simulink model "ShipSim2"  (R2022a)
settings: Solver=VariableStepAuto  StartTime=0.0  StopTime=50000.0  RelTol=1e-3
libraries: mssSimulink x1
settings Model: Creator=ADMIN  LastModifiedBy=ADMIN

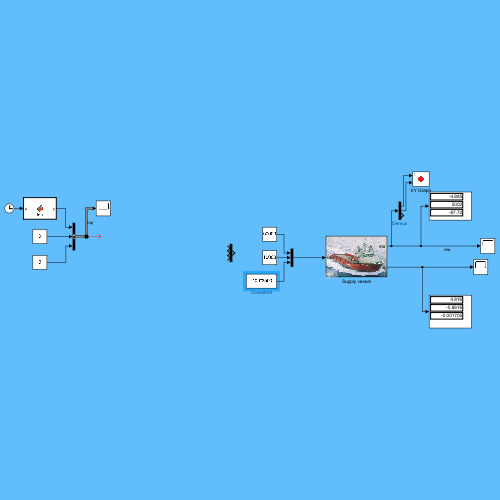
[thumbnail: Simulink's stored preview of the top-level diagram]
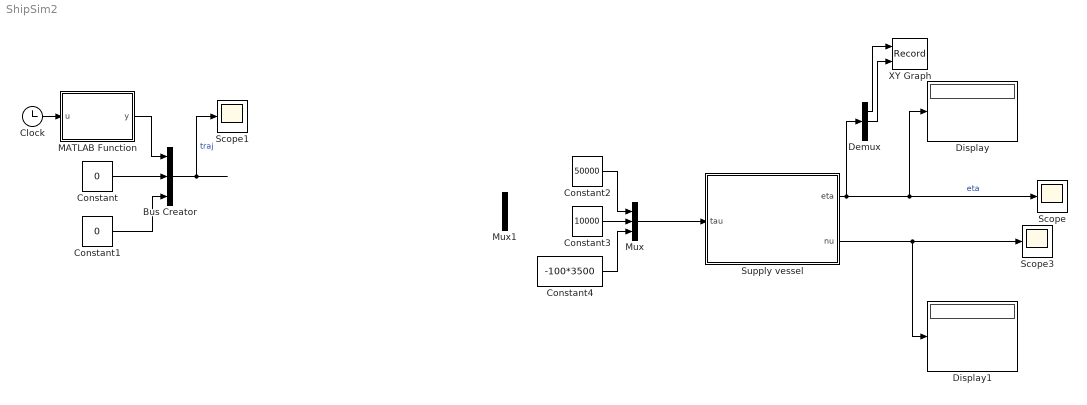
== system ShipSim2 ==
  Bus Creator : BusCreator  Inputs=3
  Clock : Clock
      settings: Decimation=50
  Constant : Constant  Value=0
  Constant1 : Constant  Value=0
  Constant2 : Constant  Value=50000
  Constant3 : Constant  Value=10000
  Constant4 : Constant  Value=-100*3500
  Demux : Demux  Outputs=3
  Display : Display
  Display1 : Display
  MATLAB Function : MATLAB Function  TreatAsAtomicUnit=on
  Mux : Mux  Inputs=3
  Mux1 : Mux  Inputs=3
  Scope : Scope
  Scope1 : Scope
  Scope3 : Scope
  Supply vessel : Subsystem  AncestorBlock=mssSimulink/Marine craft models/Supply vessel  mask(Supply Vessel (surge, sway and yaw)){D=[5.0242e4 0 0; 0 2.7229e5 -4.3933e6; 0 -4.3933e6 4.1894e8], Minv=inv( [5.3122e6 0 0; 0 8.2831e6 0; 0 0 3.7454e9] )}
      mask prompts: D "Linear damping matrix: D"; Minv "Inverse inertia matrix: Minv"
      mask help:
      | DP model
      |
      | Inputs:
      |
      |    tau = 3 DOF control input vector (generalized force)
      |
      | Outputs:
      |
      |    eta = [x, y, psi]'
      |    nu  = [u, v, r]'
      mask Display:
      | image(imread('simulink/figs/supply.jpg'))
      | color('black'); port_label('output', 1, 'eta')
      | color('black'); port_label('output', 2, 'nu')
      | color('black'); port_label('input', 1, 'tau')
  XY Graph : Record  FileSettingsInternal="{\"entries\":[{\"content\":{\"excelSettings\":{\"content\":{},\"type\":\"Streamout.ExcelSettings\"}},\"type\":\"Streamout.FileSettingStorage\",\"uuid\":\"1ec113a0-ed55-4165-962c-55b1411d3cfe\"}],\"packageUris\":[\"http://schema.mathworks.com/mf0/streamout_blocks/R2020a\"],\"version\":\"1.0\"}"  Layout=[1 1]  SignalsInternal="{\"entries\":[{\"content\":{\"signals\":[{\"content\":{\"blockPath\":[\"ShipSim2/XY Graph\"],\"channel\":[],\"dimensions\":[1],\"domain\":\"ShipSim2/XY Graph\",\"lineColor\":\"#a2142f\",\"plots\":[1],\"port\":1,\"sid\":[\"\"],\"signalID\":249,\"signalName\":\"Demux:1\"},\"type\":\"RecordBlkView.Signal\",\"uuid\":\"c85ef730-b9cc-40cf-9d67-ff760ae9bcc9\"},{\"content\":{\"blockPath\":[\"ShipSim2/XY Graph\"],\"channel\":[],\"dimensions\":[1],\"domain\":\"ShipSim2/XY Graph\",\"lineColor\":\"#139fff\",\"plots\":[1],\"port\":2,\"sid\":[\"\"],\"signalID\":253,\"signalName\":\"Demux:2\"},\"type\":\"RecordBlkView.Signal\",\"uuid\":\"b25d4ea5-1943-414a-b169-4ba9fa47959e\"}]},\"type\":\"RecordBlkView.InputSignals\",\"uuid\":\"a3917937-57db-4413-815d-85014e74e93b\"}],\"packageUris\":[\"http://schema.mathworks.com/mf0/streamout_blocks/R2020a\"],\"version\":\"1.0\"}"  VisualizationBindings="{\"xyplotplugin\":{\"info\":[{\"series\":[{\"bindingParametersList\":[{\"parameter\":\"X-Axis\",\"signalID\":249,\"signalName\":\"Demux:1\"},{\"parameter\":\"Y-Axis\",\"signalID\":253,\"signalName\":\"Demux:2\"}],\"seriesID\":61715}],\"subplotID\":1}]}}"  CompatibilityTag=XY
  wires:
  Supply vessel/1(eta) -> Demux/1, Display/1, Scope/1  "eta"
  Clock/1 -> MATLAB Function/1(u)
  MATLAB Function/1(y) -> Bus Creator/1
  Bus Creator/1 -> Scope1/1  "traj"
  Constant/1 -> Bus Creator/2
  Constant1/1 -> Bus Creator/3
  Constant3/1 -> Mux/2
  Constant2/1 -> Mux/1
  Constant4/1 -> Mux/3
  Supply vessel/2(nu) -> Display1/1, Scope3/1
  Mux/1 -> Supply vessel/1(tau)
  Demux/1 -> XY Graph/1
  Demux/2 -> XY Graph/2

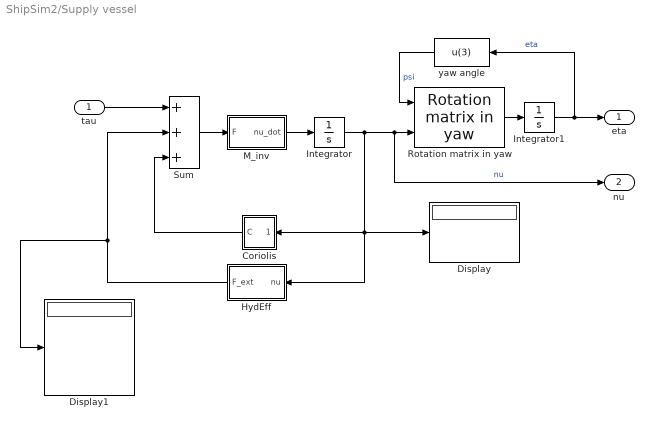
== system ShipSim2/Supply vessel ==
  tau : Inport
  Coriolis : Subsystem
  Display : Display
  Display1 : Display
  HydEff : Subsystem
  Integrator : Integrator  InitialCondition=[0 2 0]
  Integrator1 : Integrator
  M_inv : Subsystem
  "Rotation matrix in yaw " : mssSimulink/Modelling/Kinematics/Rotation matrix in yaw 
  Sum : Sum  Inputs=+++  InputSameDT=on  SaturateOnIntegerOverflow=on  OutDataTypeStr=Inherit: Same as first input
  yaw angle : Fcn  Expr=u(3)
  eta : Outport  InitialOutput=0  VectorParamsAs1DForOutWhenUnconnected=off
  nu : Outport  Port=2  InitialOutput=0  VectorParamsAs1DForOutWhenUnconnected=off
  wires:
  Sum/1 -> M_inv/1(F)
  M_inv/1(nu_dot) -> Integrator/1
  tau/1 -> Sum/1
  "Rotation matrix in yaw "/1 -> Integrator1/1
  yaw angle/1 -> "Rotation matrix in yaw "/1  "psi"
  Integrator/1 -> Display/1, HydEff/1(nu), Coriolis/1(nu), "Rotation matrix in yaw "/2, nu/1  "nu"
  Integrator1/1 -> yaw angle/1, eta/1  "eta"
  HydEff/1(F_ext) -> Display1/1, Sum/2
  Coriolis/1(C) -> Sum/3

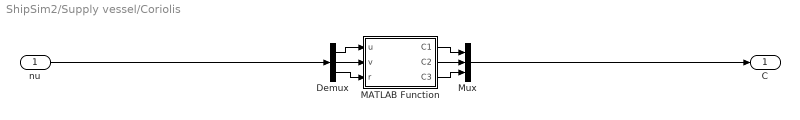
== system ShipSim2/Supply vessel/Coriolis ==
  nu : Inport
  Demux : Demux  Outputs=3
  MATLAB Function : MATLAB Function  TreatAsAtomicUnit=on
  Mux : Mux  Inputs=3
  C : Outport
  wires:
  nu/1 -> Demux/1
  MATLAB Function/2(C2) -> Mux/2
  MATLAB Function/3(C3) -> Mux/3
  MATLAB Function/1(C1) -> Mux/1
  Mux/1 -> C/1
  Demux/1 -> MATLAB Function/1(u)
  Demux/2 -> MATLAB Function/2(v)
  Demux/3 -> MATLAB Function/3(r)

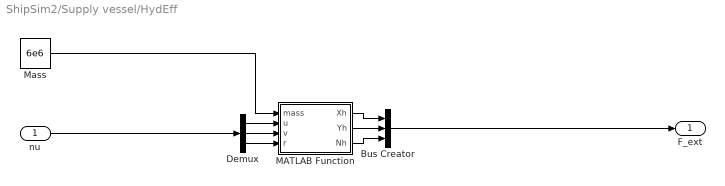
== system ShipSim2/Supply vessel/HydEff ==
  nu : Inport
  Bus Creator : BusCreator  Inputs=3
  Demux : Demux  Outputs=3
  MATLAB Function : MATLAB Function  TreatAsAtomicUnit=on
  Mass : Constant  Value=6e6
  F_ext : Outport
  wires:
  Mass/1 -> MATLAB Function/1(mass)
  MATLAB Function/1(Xh) -> Bus Creator/1
  Bus Creator/1 -> F_ext/1
  MATLAB Function/2(Yh) -> Bus Creator/2
  MATLAB Function/3(Nh) -> Bus Creator/3
  nu/1 -> Demux/1
  Demux/1 -> MATLAB Function/2(u)
  Demux/2 -> MATLAB Function/3(v)
  Demux/3 -> MATLAB Function/4(r)

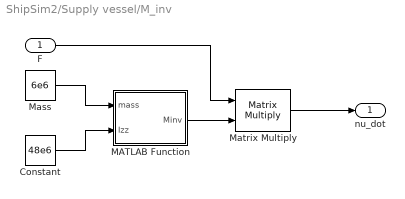
== system ShipSim2/Supply vessel/M_inv ==
  F : Inport
  Constant : Constant  Value=48e6
  MATLAB Function : MATLAB Function  TreatAsAtomicUnit=on
  Mass : Constant  Value=6e6
  Matrix Multiply : Product  Multiplication=Matrix(*)
  nu_dot : Outport
  wires:
  MATLAB Function/1(Minv) -> Matrix Multiply/2
  Mass/1 -> MATLAB Function/1(mass)
  Constant/1 -> MATLAB Function/2(Izz)
  Matrix Multiply/1 -> nu_dot/1
  F/1 -> Matrix Multiply/1

== matlab function ShipSim2/Supply vessel/Coriolis/MATLAB Function ==
  data: u input; C1 output; C2 output; C3 output; v input; r input
function [C1,    C2,    C3]    = fcn(u,v,r)

% u = nu(1);
% v = nu(2);
% r = nu(3);

x_g = 0;
m = 6e6;

C = [0                 0  -m*(x_g*r + v); ...
     0                 0             m*u; ...
     m*(x_g*r + v)  -m*u              0];

Co = C*[u;v;r];
C1 = Co(1);
C2 = Co(2);
C3 = Co(3);

end

== matlab function ShipSim2/MATLAB Function ==
  data: u input; y output
function y = fcn(u)

y = 0.5*u;

== matlab function ShipSim2/Supply vessel/M_inv/MATLAB Function ==
  data: Minv output; mass input; Izz input
function Minv = fcn(mass, Izz)

h.m   = mass;    % Mass [Kg]
h.Izz = Izz;     % Yaw Inertia
h.xG  = 0;

%%%%%%%%%%%%%%%%%%%%%%%%%%%%%%%%%%%%%%%%%%%%%%%%%%%%%%%%%%%%%%%%%%%%%%%
% The hydrodynamic derivatives are given in dimensional form, and follow
% from the original publication of Blanke and Christensen 1993.
%%%%%%%%%%%%%%%%%%%%%%%%%%%%%%%%%%%%%%%%%%%%%%%%%%%%%%%%%%%%%%%%%%%%%%%
% Data for surge equation 
h.Xudot  	= -17400.0;
h.Xuau     	= -1.96e+003;
h.Xvr    	=  0.33 * mass;
   
% Hydrodynamic coefficients in sway equation
h.Yvdot = -393000; 
h.Ypdot = -296000; 
h.Yrdot = -1400000; 
h.Yauv  = -11800; 
h.Yur   =  131000; 
h.Yvav  = -3700; 
h.Yrar  =  0;
h.Yvar  = -794000; 
h.Yrav  = -182000; 
h.Ybauv =  10800; % Y_{\phi |v u|}
h.Ybaur =  251000; 
h.Ybuu  = -74;


% Hydrodynamic coefficients in yaw equation
h.Nvdot =  538000;
h.Npdot =  0;
h.Nrdot = -38.7e6;
h.Nauv  = -92000;
h.Naur  = -4710000;
h.Nvav  =  0;
h.Nrar  = -202000000;
h.Nvar  =  0;
h.Nrav  = -15600000;
h.Nbauv = -214000;
h.Nbuar = -4980000;
h.Nbuau = -8000;
%%%%%%%%%%%%%%%%%%%%%%%%%%%%%%%%%%%%%%%%%%%%%%%%%%%%%%%%%%%%%%%%%%%%%%%%%%%


M = [(h.m-h.Xudot)                  0                  0; ...
                 0      (h.m-h.Yvdot) (h.m*h.xG-h.Yrdot); ...
                 0 (h.m*h.xG-h.Nvdot)    (h.Izz-h.Nrdot)];

Minv = inv(M);
end

== matlab function ShipSim2/Supply vessel/HydEff/MATLAB Function ==
  data: mass input; Xh output; Yh output; Nh output; u input; v input; r input
function [Xh, Yh, Nh] = fcn(mass, u, v, r)

%%%%%%%%%%%%%%%%%%%%%%%%%%%%%%%%%%%%%%%%%%%%%%%%%%%%%%%%%%%%%%%%%%%%%%%
% The hydrodynamic derivatives are given in dimensional form, and follow
% from the original publication of Blanke and Christensen 1993.
%%%%%%%%%%%%%%%%%%%%%%%%%%%%%%%%%%%%%%%%%%%%%%%%%%%%%%%%%%%%%%%%%%%%%%%
% Data for surge equation 
h.Xudot  	= -17400.0 ;
h.Xuau     	= -1.96e+003 ;
h.Xvr    	=  0.33 * mass ;
   
% Hydrodynamic coefficients in sway equation
h.Yvdot = -393000 ; 
h.Ypdot = -296000 ; 
h.Yrdot = -1400000 ; 
h.Yauv  = -11800 ; 
h.Yur   =  131000 ; 
h.Yvav  = -3700 ; 
h.Yrar   =  0 ;
h.Yvar  = -794000 ; 
h.Yrav  = -182000 ; 
h.Ybauv =  10800 ; % Y_{\phi |v u|}
h.Ybaur =  251000 ; 
h.Ybuu  = -74 ; 


% Hydrodynamic coefficients in yaw equation
h.Nvdot =  538000 ;
h.Npdot =  0 ;
h.Nrdot = -38.7e6;
h.Nauv  = -92000 ;
h.Naur  = -4710000 ;
h.Nvav  =  0 ;
h.Nrar  = -202000000 ;
h.Nvar  =  0 ;
h.Nrav  = -15600000 ;
h.Nbauv = -214000 ;
h.Nbuar = -4980000 ;
h.Nbuau = -8000 ;
%%%%%%%%%%%%%%%%%%%%%%%%%%%%%%%%%%%%%%%%%%%%%%%%%%%%%%%%%%%%%%%%%%%%%%%%%%%

au = abs(u);
av = abs(v); 
ar = abs(r);
b = 0;

% Hydrodynamic forces without added mass terms (considered in the M matrix)
Xh  = h.Xuau*u*au+h.Xvr*v*r;

Yh = h.Yauv*au*v + h.Yur*u*r + h.Yvav*v*av + h.Yvar*v*ar + h.Yrav*r*av ...
   + h.Ybauv*b*abs(u*v) + h.Ybaur*b*abs(u*r) + h.Ybuu*b*u^2;

Nh = h.Nauv*au*v + h.Naur*au*r + h.Nrar*r*ar + h.Nrav*r*av...
   +h.Nbauv*b*abs(u*b) + h.Nbuar*b*u*ar + h.Nbuau*b*u*au;

end
